simulink model "Biquad_IIR"  (R2020b)
settings: Solver=FixedStepDiscrete  StartTime=0.0  StopTime=Inf  RelTol=1e-3  EnableMultiTasking=on
libraries: dspsrcs4 x2, dsparch4 x1
settings Model: ModifiedByFormat=The MathWorks Inc.  Creator=The MathWorks, Inc.  LastModifiedBy=The MathWorks Inc.
settings DataIOCC: LimitDataPoints=on  SaveFormat=Array  SaveOutput=off  SignalLogging=off  DSMLogging=off  SaveTime=off  ReturnWorkspaceOutputs=off
settings OptimizationCC: DefaultParameterBehavior=Inlined  EnhancedBackFolding=on  PassReuseOutputArgsAs=Individual arguments  ZeroExternalMemoryAtStartup=off  ZeroInternalMemoryAtStartup=off  OptimizeBlockOrder=speed  DifferentSizesBufferReuse=on  OptimizationCustomize=off  EfficientTunableParamExpr=on
settings DebuggingCC: SolverPrmCheckMsg=warning  ParameterTunabilityLossMsg=error  AllowSymbolicDim=off  SFUnexpectedBacktrackingDiag=warning  SFNoUnconditionalDefaultTransitionDiag=warning  SFExecutionAtInitializationDiag=none  ArithmeticOperatorsInVariantConditions=warning
settings HardwareCC: ProdBitPerPointer=32  ProdBitPerSizeT=32  ProdBitPerPtrDiffT=32  ProdLargestAtomicFloat=None  ProdIntDivRoundTo=Undefined  ProdEndianess=Unspecified  ProdWordSize=32  ProdHWDeviceType=32-bit Generic
settings ModelReferenceCC: PropagateSignalLabelsOutOfModel=off
settings SFSimCC: SimUseLocalCustomCode=off  MATLABDynamicMemAlloc=off  CustomCodeUndefinedFunction=UseInterfaceOnly
settings RTWCC: Description=Embedded Coder  SystemTargetFile=ert.tlc  GenCodeOnly=on  TemplateMakefile=ert_default_tmf  RTWUseLocalCustomCode=off
settings CodeAppCC: ForceParamTrailComments=on  IgnoreCustomStorageClasses=off  OperatorAnnotations=on  SimulinkDataObjDesc=on  SFDataObjDesc=on  InsertBlockDesc=on
settings ERTTargetCC: GenerateSampleERTMain=on  InlinedParameterPlacement=NonHierarchical  ERTCustomFileTemplate=example_file_process.tlc
settings ConfigComp: CovMetricSettings=dw  CovSaveCumulativeToWorkspaceVar=on  CovSaveSingleToWorkspaceVar=on  CovExternalEMLEnable=off  CovSFcnEnable=off

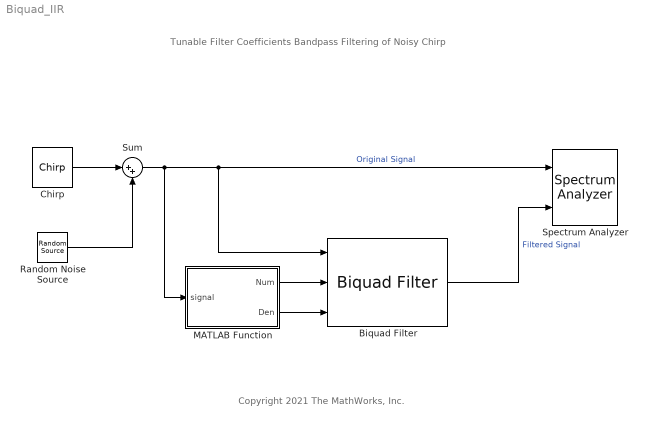
== system Biquad_IIR ==
  note: Tunable Filter Coefficients
      |
      | Bandpass Filtering of Noisy Chirp
  note: Copyright 2021 The MathWorks, Inc.
  Biquad Filter : dsparch4/Biquad Filter  FilterSource=Input port(s)  CoeffSource=Specify via dialog  FilterObject=BQF  IIRFiltStruct=Direct form II transposed  BiQuadCoeffs=[0.125869297016915377 0 -0.125869297016915377 1 -1.34390546472826866 0.915040749018974031;0.0656121180375594387 0 -0.0656121180375594387 1 -1.16122268541534979 0.905887423904348066;0.0849285957057947793 0 -0.0849285957057947793 1 -1.27123473799067255 0.870050693199404312;0.0185985573206114384 0 -0.0185985573206114384 1 -1.18347367375318724 0.863601262984001083;0.159605087222613434 0 -0.159605087222613434 1 -1.41043725076161142 0.981451841259691315;0.0600295830172420594 0 -0.0600295830172420594 1 -1.18035427365937795 0.978832212264976409;0.131232435799951502 0 -0.131232435799951502 1 -1.30744608465992096 0.889179780611041748;0.0897246573019889332 0 -0.0897246573019889332 1 -1.16761887258936792 0.880233509308278705;0.0757281400770927343 0 -0.0757281400770927343 1 -1.2371804000830291 0.85884235496636685;0.0366761055638505154 0 -0.0366761055638505154 1 -1.20726901956567767 0.856499733572212874;0.145182340958319667 0 -0.145182340958319667 1 -1.37880997391524152 0.94628865549389285;0.700444398540468249 0 -0.700444398540468249 1 -1.1653322667715198 0.939384311325326515]  ScaleValues=[0.0604683256900894403;1;1;1;1;1;1;1;1;1;1;1;1]  IC=0  ICnum=0  ICden=0  a0Flag=Warning  optimizeScaleValues=on  ScaleValueMode=Assume all are unity and optimize  InputProcessing=Columns as channels (frame based)  roundingMode=Floor  overflowMode=off  scaleValueFracLength=14  denProdOutputFracLength=30  denAccumFracLength=30  secondMemoryFracLength=15
  Chirp : dspsrcs4/Chirp  sweep=Linear  mode=Bidirectional  f0=5000  f1=8000  t1=30  Tsweep=30  phase=0  Ts=1/44100  spf=1024  datatype=Double  OutputFrames=off
      settings: SourceProductName=DSP System Toolbox
  MATLAB Function : MATLAB Function  TreatAsAtomicUnit=on
  Random Noise Source : dspsrcs4/Random Source  SrcType=Gaussian  NormMethod=Ziggurat  CltLength=12  MinVal=0  MaxVal=1  MeanVal=0  VarVal=1e-5  RepMode=Specify seed  rawSeed=3  IsInherit=off  SampMode=Discrete  SampTime=1/44100  SampFrame=1024  DataType=Double  OutComplex=Real  OutputFrames=off
  Spectrum Analyzer : SpectrumAnalyzer  NumInputPorts=2
  Sum : Sum  Inputs=|++
  wires:
  Sum/1 -> MATLAB Function/1(signal), Biquad Filter/1, Spectrum Analyzer/1  "Original Signal"
  Chirp/1 -> Sum/1
  Random Noise Source/1 -> Sum/2
  Biquad Filter/1 -> Spectrum Analyzer/2  "Filtered Signal"
  MATLAB Function/1(Num) -> Biquad Filter/2
  MATLAB Function/2(Den) -> Biquad Filter/3

== matlab function Biquad_IIR/MATLAB Function ==
  data: signal input; Num output; Den output
% Copyright 2021 The MathWorks, Inc.

function [Num, Den]= Coeffs(signal)
Fs = 44100; % Sampling Rate of Original Signal
Fn = Fs/2; % Nyquist Frequency

[pxx, f] = pwelch(signal,500,300,500,Fs); % Obtain Welch's overlapped segment averaging PSD
                                          % estimate of the signal
[~,idx] = max(pxx);

temp = f(idx);
Fc = temp(1);

peakFreq = Fc/Fn; % Peak frequency

wo = [0 peakFreq 1]; % Center frequencies
bw = [(peakFreq*0.31+0.39) 1250/Fn 0.4717]; % Filter Bandwidths (Hz)
N = [8 8 8]; % Filter Orders
G = [-60 55 -60]; % Gains

[Num, Den] = designParamEQ(N, G, wo, bw);


end
